simulink model "integrated_system_soln"  (R2018a)
settings: Solver=VariableStepAuto  StartTime=0.0  StopTime=inf  RelTol=1e-3
PreLoadFcn:
  | initParams;
values from neighbouring files (symbols this model uses):
  C = centroid(mIdx,:)    [detectGreenBall.m]
undefined symbols (not defined in the file or in its folder): none, videoinput
libraries: imaqlib x1, visionsinks x1, visiontextngfix x1
settings Model: Creator=cdsouza  LastModifiedBy=scastro

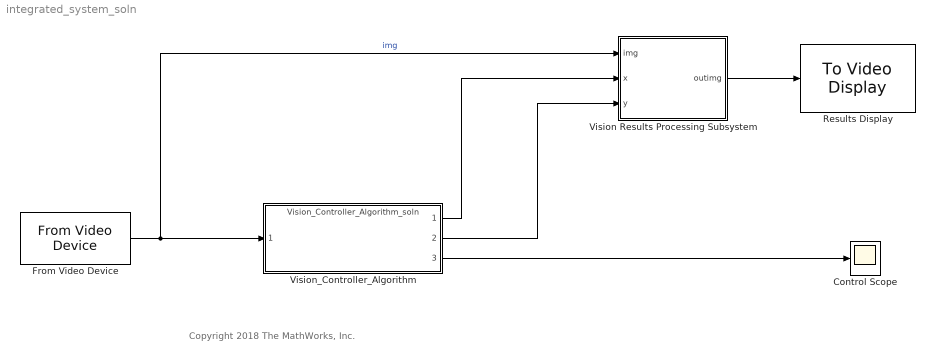
== system integrated_system_soln ==
  note: Copyright 2018 The MathWorks, Inc.
  Control Scope : Scope
  From Video Device : imaqlib/From Video Device  DeviceMenu=(none)  Device=winvideo 1 (Integrated Camera)  ObjConstructor=videoinput('winvideo', 1)  VideoFormatMenu=(none)  VideoFormat=RGB24_320x240  VideoSource=input1  ROIPosition=[0 0 240 320]  EnableHWTrigger=off  TriggerConfiguration=none/none  SampleTime=0.05  OutputPortsMode=One multidimensional signal  DataType=uint8  CanDoHWTrigger=no  ReturnedColorSpace=rgb  BlockHandle=1074.0005  ROIWidth=320  ROIHeight=240  ROIColumn=0  ROIRow=0  EngXMLPath=C:\Program Files\MATLAB\R2018a\toolbox\imaq\imaq\private  DevXMLPath=C:\ProgramData\MATLAB\SupportPackages\R2018a\toolbox\imaq\supportpackages\genericvideo\adaptor\win64  EngLibPath=C:\Program Files\MATLAB\R2018a\toolbox\imaq\imaqblks\imaqmex\win64  ColorSpace=rgb  BayerSensorAlignment=grbg
      settings: SourceProductName=Image Acquisition Toolbox
  Results Display : visionsinks/To Video Display  windowSizeMode=Normal  openAtMdlStart=on  fullScreen=off  videoWindowX=692  videoWindowY=289  saveWindowSize=off  videoWindowWidth=683  videoWindowHeight=513  inputColorFormat=RGB  inputType=Obsolete  imagePorts=One multidimensional signal  OutputDevice=On-screen video monitor  dataOrg=Column-major  isWindowOpen=off
      settings: SourceProductName=Computer Vision System Toolbox
  Vision Results Processing Subsystem : Subsystem
  Vision_Controller_Algorithm : ModelReference  ModelNameDialog=Vision_Controller_Algorithm_soln  SimulationMode=Normal  ModelReferenceVersion=1.40
  wires:
  Vision Results Processing Subsystem/1(outimg) -> Results Display/1
  From Video Device/1 -> Vision_Controller_Algorithm/1, Vision Results Processing Subsystem/1(img)  "img"
  Vision_Controller_Algorithm/1 -> Vision Results Processing Subsystem/2(x)
  Vision_Controller_Algorithm/2 -> Vision Results Processing Subsystem/3(y)
  Vision_Controller_Algorithm/3 -> Control Scope/1

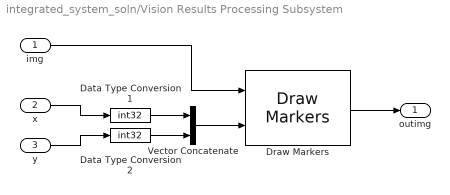
== system integrated_system_soln/Vision Results Processing Subsystem ==
  img : Inport
  x : Inport  Port=2
  y : Inport  Port=3
  Data Type Conversion1 : DataTypeConversion  OutDataTypeStr=int32
  Data Type Conversion2 : DataTypeConversion  OutDataTypeStr=int32
  Draw Markers : visiontextngfix/Draw Markers  shape=Circle  size=3  fill=off  fillClrSource=Specify via dialog  display=Black  intensity=200  color=[200 255 100]  opacity=0.6  viewport=Entire image  antialiasing=off  inType=Obsolete  imagePorts=One multidimensional signal  prodOutputMode=Binary point scaling  prodOutputWordLength=32  prodOutputFracLength=14  memoryMode=Specify word length  memoryWordLength=16  memoryFracLength=15  roundingMode=Floor  overflowMode=off
      settings: SourceProductName=Computer Vision System Toolbox  SourceProductBaseCode=VP
  Vector Concatenate : Concatenate
  outimg : Outport
  wires:
  img/1 -> Draw Markers/1
  Vector Concatenate/1 -> Draw Markers/2
  Data Type Conversion2/1 -> Vector Concatenate/2
  Draw Markers/1 -> outimg/1
  Data Type Conversion1/1 -> Vector Concatenate/1
  y/1 -> Data Type Conversion2/1
  x/1 -> Data Type Conversion1/1
